simulink model "fuzzy_rules_ani"  (R2022b)
settings: Solver=VariableStepAuto  StartTime=0.0  StopTime=10  MinStep=0.01  RelTol=1e-3
libraries: fuzblock x4, commchan3 x1
settings Model: Creator=KIIT  LastModifiedBy=KIIT
settings DebuggingCC: AlgebraicLoopMsg=error  UnconnectedInputMsg=warning  UnconnectedOutputMsg=warning  UnconnectedLineMsg=warning
settings ModelReferenceCC: EnableRefExpFcnMdlSchedulingChecks=on
settings RTWCC: DLArmComputeVersion=19.05

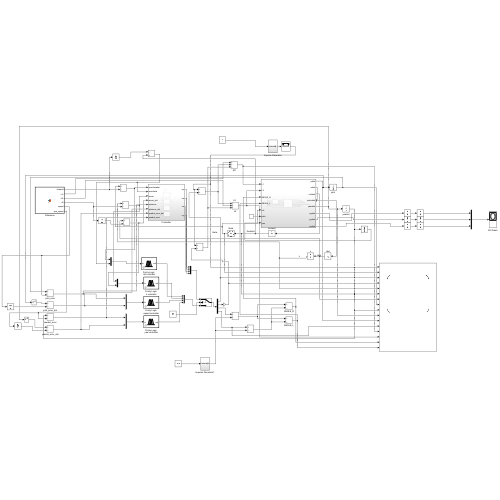
[thumbnail: Simulink's stored preview of the top-level diagram]
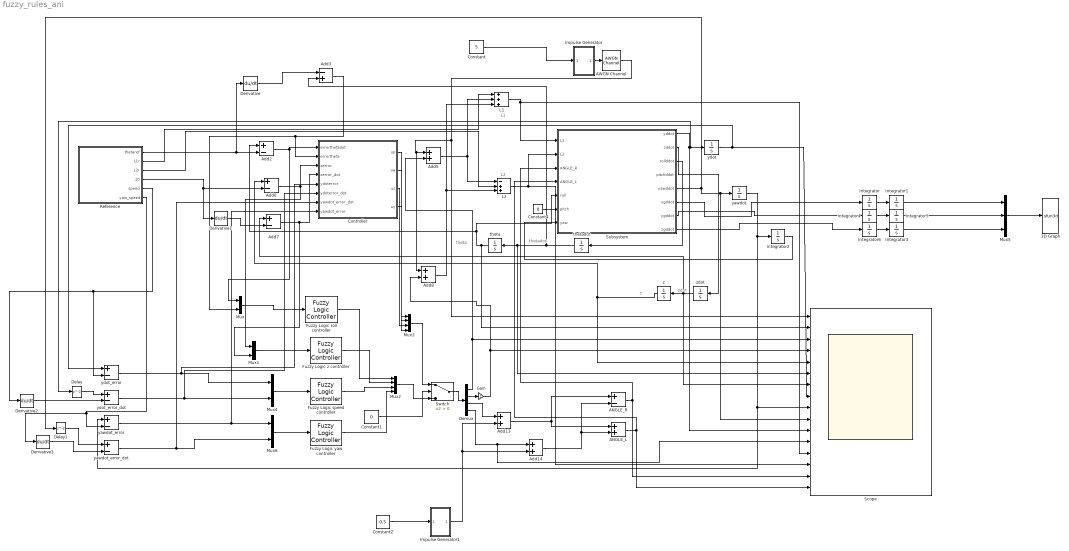
== system fuzzy_rules_ani ==
  note: z
  note: zdot
  note: L2
  note: L1
  note: theta
  note: thetadot
  3D Graph : S-Function  LoadFcn=if exist('sfun3d','file'), sfun3d([],[],[],'LoadBlock'); end  FunctionName=sfun3d  Parameters=ax,T,np,cp,gd,ls,mk,mx,hd,tb  SFunctionDeploymentMode=off  EnableBusSupport=off  mask(3D Graph){np=1, ax=[-50 50 -50 50 -50 50], mx=1e4, T=0.1, cp=[50 50 50], gd=on, hd=off, tb=off, ls=-, mk=none}
      mask prompts: np "Number of moving points (lines)"; ax "Range: [xmin xmax  ymin ymax zmin zmax]"; mx "Max number of points in each line"; T "Sampling Time"; cp "Camera position (use [0 0 1] for 2D XY view)"; gd "Grid (on|off)"; hd "HeadMarkers (on|off)"; tb "Toolbar (on|off)"; ls "LineStyle"; mk "LineMarker"
      mask help:
      | This block plots the position of several points in the XYZ space. The input contains the coordinates of all the points (x1,y1,z1,x2,y2,z2,...).
      | The number of moving points (lines), the XYZ ranges, sampling time, camera position, and grid (among other things) can be set as mask parameters.
      settings: CopyFcn=if exist('sfun3d','file'), sfun3d([],[],[],'CopyBlock'); end  DeleteFcn=if exist('sfun3d','file'), sfun3d([],[],[],'DeleteBlock'); end  NameChangeFcn=if exist('sfun3d','file'), sfun3d([],[],[],'NameChange'); end
      mask Help:
      | This block plots the position of several points in the XYZ space. The input contains the coordinates of all the points (x1,y1,z1,x2,y2,z2,...).
      | The number of moving points (lines), the XYZ ranges, sampling time, camera position, and grid (among other things) can be set as mask parameters.
      mask TypeOptions ls: - | -- | : | -. | none
      mask TypeOptions mk: none | . | + | o | * | x | square | diamond | v | ^ | > | < | pentagram | hexagram
      mask Display: plot([.05 .95 .95 .05 .05],[.45 .45 .95 .95 .45], 0.5+cos(0:0.1:2*pi)*0.3,0.7+sin(0:0.1:2*pi)*0.2)
  ANGLE_L : Sum
  ANGLE_R : Sum  Inputs=+-
  AWGN Channel : commchan3/AWGN Channel  InputProcessing=Columns as channels (frame based)  seed=67  noiseMode="Signal to noise ratio  (SNR)"  EbNodB=10  EsNodB=10  SNRdB=25  bitsPerSym=1  Ps=1  Tsym=1  variance=1
  Add{5,8,13..14} (4 alike) : Sum
  Add2 : Sum  Inputs=+-
  Add3 : Sum  Inputs=-+
  Add6 : Sum  Inputs=+-
  Add7 : Sum  Inputs=+-
  Constant : Constant  Value=5
  Constant1 : Constant  Value=0
  Constant2 : Constant  Value=0.5
  Constant4 : Constant  Value=0
  Controller : Subsystem
  Delay : Delay
  Delay1 : Delay
  Demux : Demux
  Derivative{,1..3} (4 alike) : Derivative
  Fuzzy Logic roll controller : fuzblock/Fuzzy Logic  Controller  FIS=fuzzy_rules_ani  OutputSampleNumber=101  DataType=double  FuzzifiedInputs=off  RuleFiringStrengths=off  RuleOutputs=off  AggregatedOutputs=off  SimulateUsing=Interpreted execution  OutOfRangeInputValueMessage=warning  NoRuleFiredMessage=warning  EmptyOutputFuzzySetMessage=warning
  Fuzzy Logic speed controller : fuzblock/Fuzzy Logic  Controller  FIS=fuzzy_y_rules_ani  OutputSampleNumber=101  DataType=double  FuzzifiedInputs=off  RuleFiringStrengths=off  RuleOutputs=off  AggregatedOutputs=off  SimulateUsing=Interpreted execution  OutOfRangeInputValueMessage=warning  NoRuleFiredMessage=warning  EmptyOutputFuzzySetMessage=warning
  Fuzzy Logic yaw controller : fuzblock/Fuzzy Logic  Controller  FIS=fuzzy_yaw_rules_ani  OutputSampleNumber=101  DataType=double  FuzzifiedInputs=off  RuleFiringStrengths=off  RuleOutputs=off  AggregatedOutputs=off  SimulateUsing=Interpreted execution  OutOfRangeInputValueMessage=warning  NoRuleFiredMessage=warning  EmptyOutputFuzzySetMessage=warning
  Fuzzy Logic z controller : fuzblock/Fuzzy Logic  Controller  FIS=fuzzy_z_rules_ani  OutputSampleNumber=101  DataType=double  FuzzifiedInputs=off  RuleFiringStrengths=off  RuleOutputs=off  AggregatedOutputs=off  SimulateUsing=Interpreted execution  OutOfRangeInputValueMessage=warning  NoRuleFiredMessage=warning  EmptyOutputFuzzySetMessage=warning
  Gain : Gain
  Impulse Generator : Subsystem
  Impulse Generator1 : Subsystem
  Integrator{,1..6} (7 alike) : Integrator
  L1 : Sum  Inputs=+++
  L2 : Sum  Inputs=-++
  Mux{,1,4,6} (4 alike) : Mux  Inputs=2
  Mux2 : Mux
  Mux3 : Mux
  Mux5 : Mux  Inputs=3
  Reference : MATLAB Function  TreatAsAtomicUnit=on
  Scope : Scope  NumInputPorts=16
  Subsystem : Subsystem
  Switch : Switch  Criteria=u2 > Threshold  SaturateOnIntegerOverflow=off  InputSameDT=off
  theta : Integrator  WrapState=on
  thetadot : Integrator
  yawdot : Integrator  InitialCondition=3
  yawdot_error : Sum  Inputs=+-
  yawdot_error_dot : Sum  Inputs=+-
  ydot : Integrator
  ydot_error : Sum  Inputs=+-
  ydot_error_dot : Sum  Inputs=+-
  z : Integrator
  zdot : Integrator
  wires:
  Reference/2(L1r) -> L1/1
  Reference/3(L2r) -> L2/2
  L1/1 -> Scope/13, Subsystem/1(L1)
  L2/1 -> Scope/14, Subsystem/2(L2)
  Subsystem/3(rollddot) -> thetadot/1
  thetadot/1 -> Add3/2, Scope/6, theta/1
  theta/1 -> Scope/2, Subsystem/5(roll), Add2/1
  Reference/1(thetaref) -> Add2/2, Derivative/1
  Derivative/1 -> Add3/1
  Add5/1 -> L1/2, L2/1
  Subsystem/2(zddot) -> zdot/1
  zdot/1 -> Scope/7, Add7/1, z/1
  Reference/4(z0) -> Derivative1/1, Add6/2
  z/1 -> Add6/1, Scope/5
  Derivative1/1 -> Add7/2
  Add8/1 -> L1/3, L2/3
  AWGN Channel/1 -> Scope/1, Add8/1, Add5/1
  Add6/1 -> Mux1/1, Controller/3(zerror)
  Add7/1 -> Controller/4(zerror_dot), Mux1/2
  Mux/1 -> Fuzzy Logic roll controller/1
  Constant/1 -> Impulse Generator/1(Intensity)
  Mux1/1 -> Fuzzy Logic z controller/1
  Add3/1 -> Controller/2(errortheta), Mux/2
  Add2/1 -> Mux/1, Controller/1(errorthetadot)
  Fuzzy Logic z controller/1 -> Mux2/2
  Fuzzy Logic roll controller/1 -> Mux2/1
  Mux2/1 -> Switch/3
  Switch/1 -> Demux/1
  Demux/1 -> Add5/2, Scope/3
  Gain/1 -> Add8/2, Scope/4
  Controller/1(up) -> Mux3/1
  Controller/2(ua) -> Mux3/2
  Mux3/1 -> Switch/1
  Constant1/1 -> Switch/2
  ANGLE_R/1 -> Subsystem/3(ANGLE_R), Scope/15
  Integrator2/1 -> Subsystem/7(yaw)
  Constant4/1 -> Subsystem/6(pitch)
  Demux/2 -> Gain/1
  Subsystem/1(yddot) -> Scope/11, Delay/1, ydot/1
  Controller/3(us) -> Mux3/3
  Controller/4(uy) -> Mux3/4
  Fuzzy Logic speed controller/1 -> Mux2/3
  Fuzzy Logic yaw controller/1 -> Mux2/4
  Add13/1 -> ANGLE_R/1, ANGLE_L/1
  Add14/1 -> ANGLE_R/2, ANGLE_L/2
  ydot_error_dot/1 -> Controller/6(ydoterror_dot), Mux4/2
  ydot_error/1 -> Controller/5(ydoterror), Mux4/1
  Mux4/1 -> Fuzzy Logic speed controller/1
  yawdot_error_dot/1 -> Controller/7(yawdot_error_dot), Mux6/2
  yawdot_error/1 -> Controller/8(yawdot_error), Mux6/1
  Mux6/1 -> Fuzzy Logic yaw controller/1
  ANGLE_L/1 -> Subsystem/4(ANGLE_L), Scope/16
  ydot/1 -> ydot_error/1, Scope/8
  Reference/5(speed) -> Derivative2/1, ydot_error/2
  Derivative2/1 -> ydot_error_dot/2
  Derivative3/1 -> yawdot_error_dot/2
  Subsystem/5(yawddot) -> Scope/10, yawdot/1, Delay1/1
  yawdot/1 -> Integrator2/1, yawdot_error/1, Scope/9
  Reference/6(yaw_speed) -> Derivative3/1, yawdot_error/2
  Demux/3 -> Add13/1
  Demux/4 -> Scope/12, Add14/1
  Delay/1 -> ydot_error_dot/1
  Delay1/1 -> yawdot_error_dot/1
  Impulse Generator1/1(Out1) -> Add14/2, Add13/2
  Constant2/1 -> Impulse Generator1/1(Intensity)
  Subsystem/6(xgddot) -> Integrator/1
  Integrator/1 -> Integrator1/1
  Subsystem/7(ygddot) -> Integrator4/1
  Integrator4/1 -> Integrator5/1
  Subsystem/8(zgddot) -> Integrator6/1
  Integrator6/1 -> Integrator3/1
  Impulse Generator/1(Out1) -> AWGN Channel/1
  Integrator5/1 -> Mux5/2
  Integrator3/1 -> Mux5/3
  Integrator1/1 -> Mux5/1
  Mux5/1 -> 3D Graph/1

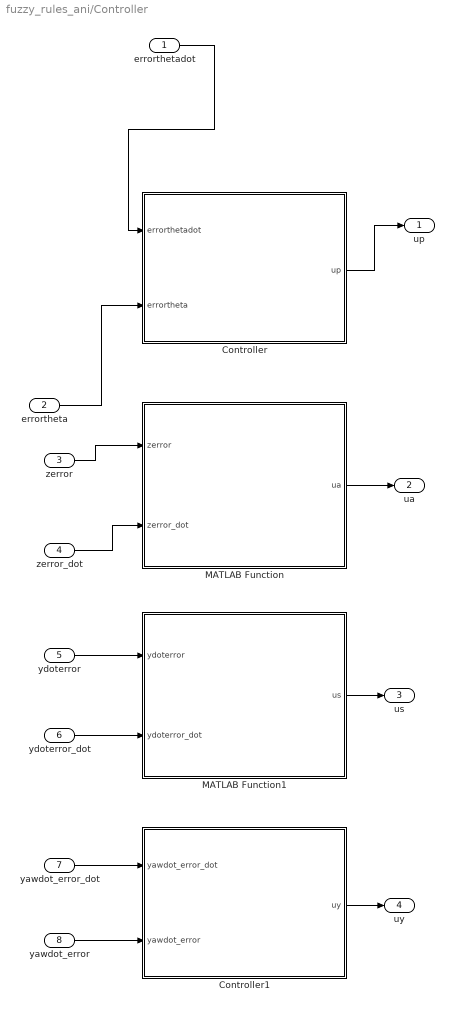
== system fuzzy_rules_ani/Controller ==
  errorthetadot : Inport
  errortheta : Inport  Port=2
  zerror : Inport  Port=3
  zerror_dot : Inport  Port=4
  ydoterror : Inport  Port=5
  ydoterror_dot : Inport  Port=6
  yawdot_error_dot : Inport  Port=7
  yawdot_error : Inport  Port=8
  Controller : MATLAB Function  TreatAsAtomicUnit=on
  Controller1 : MATLAB Function  TreatAsAtomicUnit=on
  MATLAB Function : MATLAB Function  TreatAsAtomicUnit=on
  MATLAB Function1 : MATLAB Function  TreatAsAtomicUnit=on
  up : Outport
  ua : Outport  Port=2
  us : Outport  Port=3
  uy : Outport  Port=4
  wires:
  errortheta/1 -> Controller/2(errortheta)
  MATLAB Function/1(ua) -> ua/1
  errorthetadot/1 -> Controller/1(errorthetadot)
  zerror/1 -> MATLAB Function/1(zerror)
  Controller/1(up) -> up/1
  zerror_dot/1 -> MATLAB Function/2(zerror_dot)
  Controller1/1(uy) -> uy/1
  MATLAB Function1/1(us) -> us/1
  ydoterror/1 -> MATLAB Function1/1(ydoterror)
  ydoterror_dot/1 -> MATLAB Function1/2(ydoterror_dot)
  yawdot_error_dot/1 -> Controller1/1(yawdot_error_dot)
  yawdot_error/1 -> Controller1/2(yawdot_error)

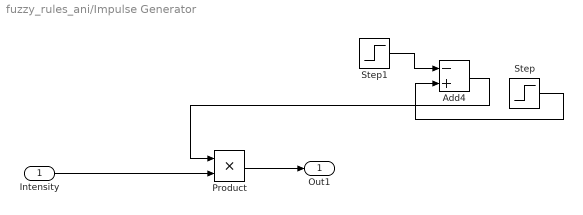
== system fuzzy_rules_ani/Impulse Generator ==
  Intensity : Inport
  Add4 : Sum  Inputs=-+
  Product : Product
  Step : Step  SampleTime=0
  Step1 : Step  Time=2  SampleTime=0
  Out1 : Outport
  wires:
  Step1/1 -> Add4/1
  Step/1 -> Add4/2
  Add4/1 -> Product/1
  Product/1 -> Out1/1
  Intensity/1 -> Product/2

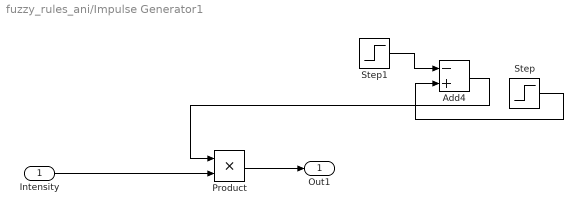
== system fuzzy_rules_ani/Impulse Generator1 ==
  Intensity : Inport
  Add4 : Sum  Inputs=-+
  Product : Product
  Step : Step  SampleTime=0
  Step1 : Step  Time=1.5  SampleTime=0
  Out1 : Outport
  wires:
  Step1/1 -> Add4/1
  Step/1 -> Add4/2
  Add4/1 -> Product/1
  Product/1 -> Out1/1
  Intensity/1 -> Product/2

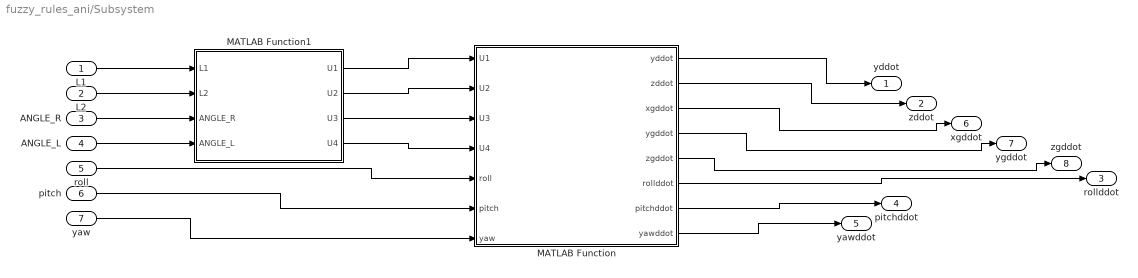
== system fuzzy_rules_ani/Subsystem ==
  L1 : Inport
  L2 : Inport  Port=2
  ANGLE_R : Inport  Port=3
  ANGLE_L : Inport  Port=4
  roll : Inport  Port=5
  pitch : Inport  Port=6
  yaw : Inport  Port=7
  MATLAB Function : MATLAB Function  TreatAsAtomicUnit=on
  MATLAB Function1 : MATLAB Function  TreatAsAtomicUnit=on
  yddot : Outport
  zddot : Outport  Port=2
  rollddot : Outport  Port=3
  pitchddot : Outport  Port=4
  yawddot : Outport  Port=5
  xgddot : Outport  Port=6
  ygddot : Outport  Port=7
  zgddot : Outport  Port=8
  wires:
  MATLAB Function1/1(U1) -> MATLAB Function/1(U1)
  MATLAB Function1/2(U2) -> MATLAB Function/2(U2)
  MATLAB Function1/3(U3) -> MATLAB Function/3(U3)
  MATLAB Function1/4(U4) -> MATLAB Function/4(U4)
  L1/1 -> MATLAB Function1/1(L1)
  L2/1 -> MATLAB Function1/2(L2)
  ANGLE_R/1 -> MATLAB Function1/3(ANGLE_R)
  ANGLE_L/1 -> MATLAB Function1/4(ANGLE_L)
  roll/1 -> MATLAB Function/5(roll)
  pitch/1 -> MATLAB Function/6(pitch)
  yaw/1 -> MATLAB Function/7(yaw)
  MATLAB Function/1(yddot) -> yddot/1
  MATLAB Function/2(zddot) -> zddot/1
  MATLAB Function/6(rollddot) -> rollddot/1
  MATLAB Function/7(pitchddot) -> pitchddot/1
  MATLAB Function/8(yawddot) -> yawddot/1
  MATLAB Function/3(xgddot) -> xgddot/1
  MATLAB Function/4(ygddot) -> ygddot/1
  MATLAB Function/5(zgddot) -> zgddot/1

== matlab function fuzzy_rules_ani/Controller/MATLAB Function1 ==
  data: ydoterror input; us output; ydoterror_dot input
function us = fcn(ydoterror,ydoterror_dot)
m = 0.87;
g = 9.8;
d = 0.2;
k3 = 3;
k4 = 3;
ubar = m*((1+k3)*ydoterror+k4*ydoterror_dot);
ua = ubar/2.0;
us = atan(ua);

== matlab function fuzzy_rules_ani/Controller/Controller ==
  data: errorthetadot input; up output; errortheta input
function up  = fcn(errorthetadot, errortheta)
m = 0.87;
Iy = 0.43;
g = 9.81;
d = 0.175;
k1 = 24;
k2 = 7;
up1 = (Iy/(2*d))*((1+k1)*errortheta + k2*errorthetadot);
up = -up1;

== matlab function fuzzy_rules_ani/Reference ==
  data: thetaref output; L1r output; L2r output; z0 output; speed output; yaw_speed output
function [thetaref, L1r, L2r, z0, speed, yaw_speed] = fcn()
m = 0.87;
g = 9.81;
p = 1.225;
h = 0.085;
d = 0.175;
kt = 6.46;
Ix = 0.0043;
Iy = 0.0142;
Iz = 0.0176;
Ixz = 0.0176;
u = [0, m*g/2, m*g/2];
thetaref = 0;
L1r = m*g/2;
L2r = m*g/2;
z0 = 0;
speed = 0;
yaw_speed = 0;

== matlab function fuzzy_rules_ani/Controller/MATLAB Function ==
  data: zerror input; ua output; zerror_dot input
function ua = fcn(zerror,zerror_dot)
m = 0.87;
g = 9.8;
d = 0.175;
k3 = 3;
k4 = 3;
ubar = m*((1+k3)*zerror+k4*zerror_dot);
ua = ubar/2.0;

== matlab function fuzzy_rules_ani/Subsystem/MATLAB Function ==
  data: U1 input; U2 input; U3 input; U4 input; roll input; pitch input; yaw input; yddot output; zddot output; xgddot output; ygddot output; zgddot output; rollddot output; pitchddot output; yawddot output
function [yddot, zddot, xgddot, ygddot, zgddot, rollddot, pitchddot, yawddot] = fcn(U1, U2, U3, U4, roll, pitch, yaw)
m = 0.87;
g = 9.81;
p = 1.225;
h = 0.085;
l = 0.175;
kt = 6.46;
Ix = 0.43;
Iy = 0.0142;
Iz = 0.0176;
Ixz = 0.0176;
xgddot = (-U1*(sin(roll)*sin(yaw)+cos(roll)*sin(pitch)*cos(yaw))-U3*(cos(pitch)*cos(yaw)))/m;
ygddot = (U1*(sin(roll)*cos(yaw)-cos(roll)*sin(pitch)*sin(yaw))+U3*(cos(pitch)*sin(yaw)))/m;
zgddot = ((-U1*(cos(roll)*cos(pitch))-U3*(sin(pitch)))/m)+g;
yddot = (U3)/m;
zddot = U1/m - g;
rollddot = l*U2/Ix;
pitchddot = h*U3/Iy;
yawddot = l*U4/Iz;

== matlab function fuzzy_rules_ani/Subsystem/MATLAB Function1 ==
  data: L1 input; U1 output; L2 input; ANGLE_R input; ANGLE_L input; U2 output; U3 output; U4 output
function [U1, U2, U3, U4] = fcn(L1, L2, ANGLE_R, ANGLE_L)

U1 = L1*cos(ANGLE_L)+L2*cos(ANGLE_R);
U2 = L1*cos(ANGLE_L)-L2*cos(ANGLE_R);
U3 = L1*sin(ANGLE_L)+L2*sin(ANGLE_R);
U4 = L1*sin(ANGLE_L)-L2*sin(ANGLE_R);

== matlab function fuzzy_rules_ani/Controller/Controller1 ==
  data: yawdot_error_dot input; uy output; yawdot_error input
function uy  = fcn(yawdot_error_dot, yawdot_error)
m = 0.87;
Iy = 0.43;
Iz = 0.0176;
g = 9.81;
d = 0.175;
k1 = 24;
k2 = 7;
up1 = (Iz/(2*d))*((1+k1)*yawdot_error + k2*yawdot_error_dot);
up = -up1;
uy = atan(up);
